simulink model "GlideslopeController"  (R2021b)
settings: Solver=VariableStepAuto  StartTime=0.0  StopTime=10.0  RelTol=1e-3
values from neighbouring files (symbols this model uses):
  K_c = 1    [Glideslope.m]
  max_dev_elevator = 25 - trim_control_lo(1)    [Glideslope.m]
  max_dev_thrust = 19000 - trim_thrust_lo    [Glideslope.m]
  min_dev_elevator = -25 - trim_control_lo(1)    [Glideslope.m]
  min_dev_thrust = 1000 - trim_thrust_lo    [Glideslope.m]
  P_0 = V_0*10    (= 3000)    [Glideslope.m]
  V_0 = 300    [Glideslope.m]
  W_1 = 0.1    [Glideslope.m]
libraries: slpidlib x1, cstblocks x1
settings Model: Creator=ddefu  LastModifiedBy=ddefu

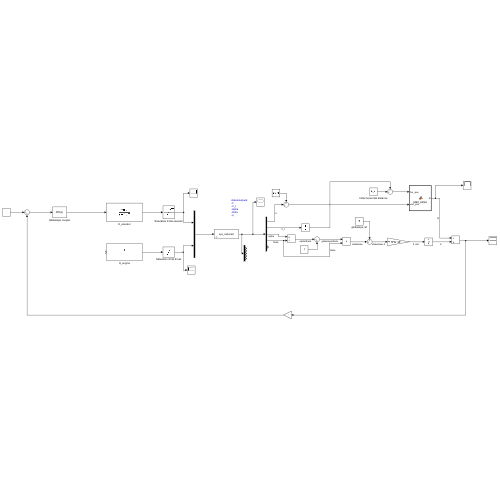
[thumbnail: Simulink's stored preview of the top-level diagram]
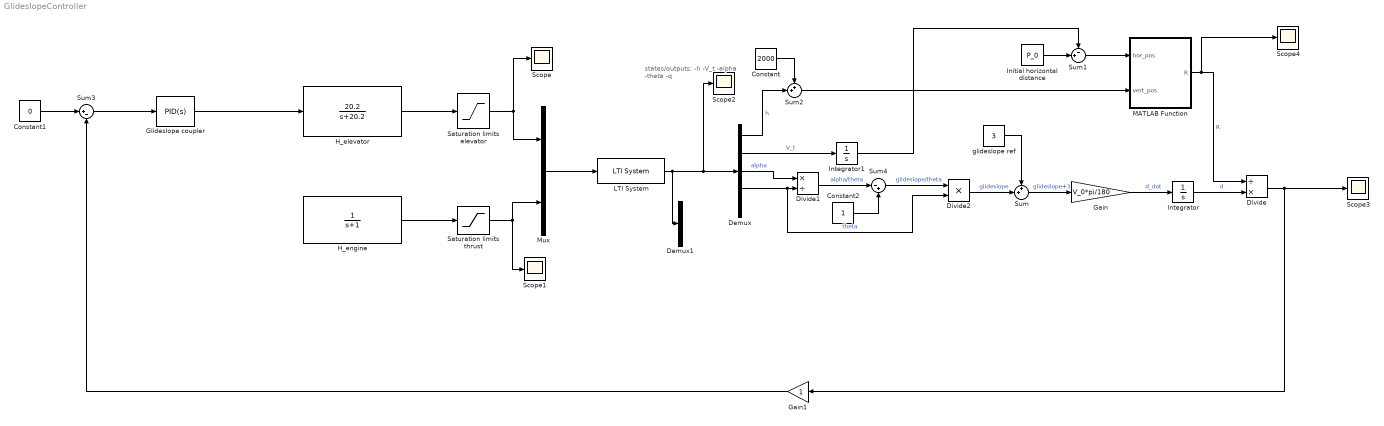
== system GlideslopeController ==
  note: states/outputs:
      | -h
      | -V_t
      | -alpha
      | -theta
      | -q
  Constant : Constant  Value=2000
  Constant1 : Constant  Value=0
  Constant2 : Constant
  Demux : Demux  Outputs=5
  Demux1 : Demux  Outputs=5
  Divide : Product  Inputs=/*
  Divide1 : Product  Inputs=*/
  Divide2 : Product  Inputs=**
  Gain : Gain  Gain=V_0*pi/180
  Gain1 : Gain
  Glideslope coupler : slpidlib/PID Controller  Controller=PID  Form=Parallel  TimeDomain=Continuous-time  UseExternalTs=off  SampleTime=-1  IntegratorMethod=Forward Euler  FilterMethod=Forward Euler  ControllerParametersSource=internal  P=K_c  I=W_1  D=0  UseFilter=on  N=100  TunerSelectOption=Transfer Function Based (PID Tuner App)  InitialConditionSource=internal  InitialConditionForIntegrator=0  InitialConditionForFilter=0  DifferentiatorICPrevScaledInput=0  ExternalReset=none  TrackingMode=off  Kt=1  LimitOutput=off  SatLimitsSource=internal  UpperSaturationLimit=inf  LowerSaturationLimit=-inf  LinearizeAsGain=on  AntiWindupMode=none  Kb=1  POutMin=[]  POutMax=[]  IOutMin=[]  IOutMax=[]  DOutMin=[]  DOutMax=[]  NOutMin=[]  NOutMax=[]  SumOutMin=[]  SumOutMax=[]  SaturationOutMin=[]  SaturationOutMax=[]  PParamMin=[]  PParamMax=[]  IParamMin=[]  IParamMax=[]  DParamMin=[]  DParamMax=[]  NParamMin=[]  NParamMax=[]  KbParamMin=[]  KbParamMax=[]  KtParamMin=[]  KtParamMax=[]  KbOutMin=[]  KbOutMax=[]  KtOutMin=[]  KtOutMax=[]  IntegratorOutMin=[]  IntegratorOutMax=[]  FilterOutMin=[]  FilterOutMax=[]  SumI1OutMin=[]  SumI1OutMax=[]  SumI2OutMin=[]  SumI2OutMax=[]  SumI3OutMin=[]  SumI3OutMax=[]  SumI4OutMin=[]  SumI4OutMax=[]  SumDOutMin=[]  SumDOutMax=[]  DifferentiatorOutMin=[]  DifferentiatorOutMax=[]  FilterDiffOutCoefMin=[]  FilterDiffOutCoefMax=[]  ReciprocalOutMin=[]  ReciprocalOutMax=[]  SumDenOutMin=[]  SumDenOutMax=[]  SumNumOutMin=[]  SumNumOutMax=[]  DivideOutMin=[]  DivideOutMax=[]  UdiffTsProdOutMin=[]  UdiffTsProdOutMax=[]  NTsProdOutMin=[]  NTsProdOutMax=[]  UintegralTsProdOutMin=[]  UintegralTsProdOutMax=[]  UngainTsProdOutMin=[]  UngainTsProdOutMax=[]  IntegratorContinuousStateAttributes=''  IntegratorStateMustResolveToSignalObject=off  IntegratorRTWStateStorageClass=Auto  FilterContinuousStateAttributes=''  FilterStateMustResolveToSignalObject=off  FilterRTWStateStorageClass=Auto  ParallelPVariant=InternalParameters  IdealPVariant=Disabled  IVariant=InternalParameters  DVariant=InternalParameters  IntegratorVariant=Continuous  SatVariant=Disabled  AWVariant=Passthrough  PCopyVariant=Disabled  TRVariant=Disabled  FdbkBlocksVariant=Forward  IdealPFdbkVariant=Disabled  SatFdbkVariant=Disabled  DerivativeFilterVariant=ContFilter  NVariant=InternalParameters  NCopyVariant=Disabled  FilterICVariant=InternalICsFilter  IntegratorICVariant=InternalICs  ExternalResetVariant=Disabled  TRSumVariant=Passthrough  SumFdbkVariant=Disabled  SumVariant=Sum_PID  TsampFilterVariant=InternalTs  TsampNgainVariant=Passthrough  TsampIntegralVariant=Passthrough  ExternalSaturationOutDataTypeStr=Inherit: Same as second input
  H_elevator : TransferFcn  Numerator=[20.2]  Denominator=[1 20.2]
  H_engine : TransferFcn  Denominator=[1 1]
  Initial horizontal distance : Constant  Value=P_0
  Integrator : Integrator
  Integrator1 : Integrator
  LTI System : cstblocks/LTI System  sys=sys_reduced  IC=[]
  MATLAB Function : MATLAB Function  TreatAsAtomicUnit=on
  Mux : Mux  Inputs=2
  Saturation limits elevator : Saturate  UpperLimit=max_dev_elevator  LowerLimit=min_dev_elevator
  Saturation limits thrust : Saturate  UpperLimit=max_dev_thrust  LowerLimit=min_dev_thrust
  Scope{,1..4} (5 alike) : Scope
  Sum : Sum  Inputs=++|
  Sum1 : Sum  Inputs=-+|
  Sum2 : Sum  Inputs=++|
  Sum3 : Sum  Inputs=|+-
  Sum4 : Sum  Inputs=|-+
  glideslope ref : Constant  Value=3
  wires:
  H_elevator/1 -> Saturation limits elevator/1
  H_engine/1 -> Saturation limits thrust/1
  Mux/1 -> LTI System/1
  Saturation limits elevator/1 -> Scope/1, Mux/1
  Saturation limits thrust/1 -> Scope1/1, Mux/2
  LTI System/1 -> Demux1/1, Scope2/1, Demux/1
  Sum4/1 -> Divide2/1  "glideslope/theta"
  glideslope ref/1 -> Sum/1
  Gain/1 -> Integrator/1  "d_dot"
  Sum/1 -> Gain/1  "glideslope+3"
  Integrator1/1 -> Sum1/1
  Initial horizontal distance/1 -> Sum1/2
  Constant/1 -> Sum2/1
  Demux/2 -> Integrator1/1  "V_t"
  Demux/1 -> Sum2/2  "h"
  Sum1/1 -> MATLAB Function/1(hor_pos)
  Sum2/1 -> MATLAB Function/2(vert_pos)
  MATLAB Function/1(R) -> Scope4/1, Divide/1  "R"
  Integrator/1 -> Divide/2  "d"
  Divide/1 -> Scope3/1, Gain1/1
  Gain1/1 -> Sum3/2
  Sum3/1 -> Glideslope coupler/1
  Constant1/1 -> Sum3/1
  Glideslope coupler/1 -> H_elevator/1
  Demux/3 -> Divide1/1  "alpha"
  Constant2/1 -> Sum4/2
  Divide1/1 -> Sum4/1  "alpha/theta"
  Demux/4 -> Divide2/2, Divide1/2  "theta"
  Divide2/1 -> Sum/2  "glideslope"

== matlab function GlideslopeController/MATLAB Function ==
  data: hor_pos input; R output; vert_pos input
function R = slant_range(hor_pos, vert_pos)

R = sqrt(hor_pos^2+vert_pos^2);
